simulink model "HopperRaibertSpeedGoat"  (R2025a)
settings: Solver=FixedStepAuto  StartTime=0.0  StopTime=inf  RelTol=1e-3
undefined symbols (not defined in the file): HS, IO291
libraries: aru_toolbox x3, speedgoatlib_IO291 x1, simulink x1
settings Model: Creator=Gavin  LastModifiedBy=user
settings SolverCC: ConcurrentTasks=on  PositivePriorityOrder=on  AutoInsertRateTranBlk=on
settings OptimizationCC: BlockReduction=off  OptimizeBlockIOStorage=off
settings DebuggingCC: TasksWithSamePriorityMsg=none
settings HardwareCC: ProdBitPerLong=64.0  ProdLongLongMode=on  ProdHWDeviceType=Intel->x86-64 (Linux 64)
settings RTWCC: SystemTargetFile=speedgoat.tlc  TemplateMakefile=slrealtime_default_tmf  Toolchain=Simulink Real-Time Toolchain  BuildConfiguration=Faster Runs  CodeExecutionProfiling=on  TargetLang=C++  Description=Speedgoat Real-Time Target Machine
settings SimulinkRealTimeTargetCC: SLRTFileLogMaxRuns=1.0  ExtModeMaxTrigDuration=10.0  ExtModeStaticAllocSize=1000000.0  ExtModeTransport=0.0  MultiwordLength=2048.0  DynamicStringBufferSize=256.0  PreserveMATLABNamespacesInGeneratedCode=on  SubcomponentCodeInterfacePackaging=Reusable function  MATLABClassNameForMDSCustomization=Simulink.SoftwareTarget.GRTCustomization  InstructionSetFMA=off  LogToMDFFile=off
settings ExplorerConfigSet: InternalSimMechanicsExplorerSettings="<ExplorerConfiguration><canonicalview>default</canonicalview><TilePanel><TileInfo><Tiles Columns=\"1\" Count=\"1\" Height=\"832\" Rows=\"1\" Width=\"1462\"><Row Weight=\"1\"/><Column Weight=\"1\"/><Tile Height=\"1\" Width=\"1\" X=\"0\" Y=\"0\"/></Tiles></TileInfo><SceneInfo><SceneViewer><IsThisViewStd><IsStandardView>off</IsStandardView><StandardViewName>Front</StandardViewName></IsThisViewStd><BGColor><R>1</R><G>1</G><B>1</B><A>1</A></BGColor><Camera><DoPerspective>on</DoPerspective><Position><X>-0.15165999999999999</X><Y>3.9971199999999998</Y><Z>0.85099999999999998</Z></Position><Center><X>0</X><Y>0</Y><Z>0.10100000000000001</Z></Center><Up><X>0.0069873130929931429</X><Y>-0.18415619748295364</Y><Z>0.98287215464899591</Z></Up><XLim>1.8977346774231529</XLim><YLim>1.8977346774231529</YLim><ViewLimDist>0.01</ViewLimDist></Camera></SceneViewer></SceneInfo></TilePanel><MechEditorPanel><GfxPanelCameraMap><MapElement CameraMLId=\"Camera1\" GfxPanelIndex=\"0\"/></GfxPanelCameraMap><Cameras><Camera><Id>Camera1</Id><Value><Name>FollowBot</Name><NativeCamera><PositionTrackingFeature>Subsystem.Half_Baleka_Simscape_WIP.Planarising_Boom.Center_to_CameraUp.F</PositionTrackingFeature><CenterTrackingFeature>Subsystem.Half_Baleka_Simscape_WIP.Planarising_Boom.Center_to_Camera.B</CenterTrackingFeature><UpVectorTrackingFeature>Subsystem.Half_Baleka_Simscape_WIP.Planarising_Boom.Center_to_Camera.B</UpVectorTrackingFeature><CenterTrackingOrigin>on</CenterTrackingOrigin><UpVectorTrackingDirection>+Y</UpVectorTrackingDirection></NativeCamera></Value></Camera></Cameras><VideoCreator><IncludeTiles>All</IncludeTiles><IncludeTime>on</IncludeTime><IncludeWorldFrame>off</IncludeWorldFrame><PlaybackSpeedRatio>1</PlaybackSpeedRatio><FrameRate>30</FrameRate><FrameSize>auto</FrameSize><VideoFormat>MotionJPEGAVI</VideoFormat></VideoCreator></MechEditorPanel><PlaybackSettings><PlaybackSpeedFactor>1</PlaybackSpeedFactor></PlaybackSettings></ExplorerConfiguration>"

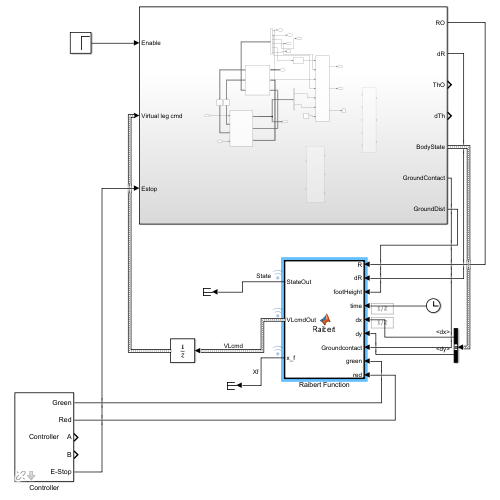
[thumbnail: Simulink's stored preview of the top-level diagram]
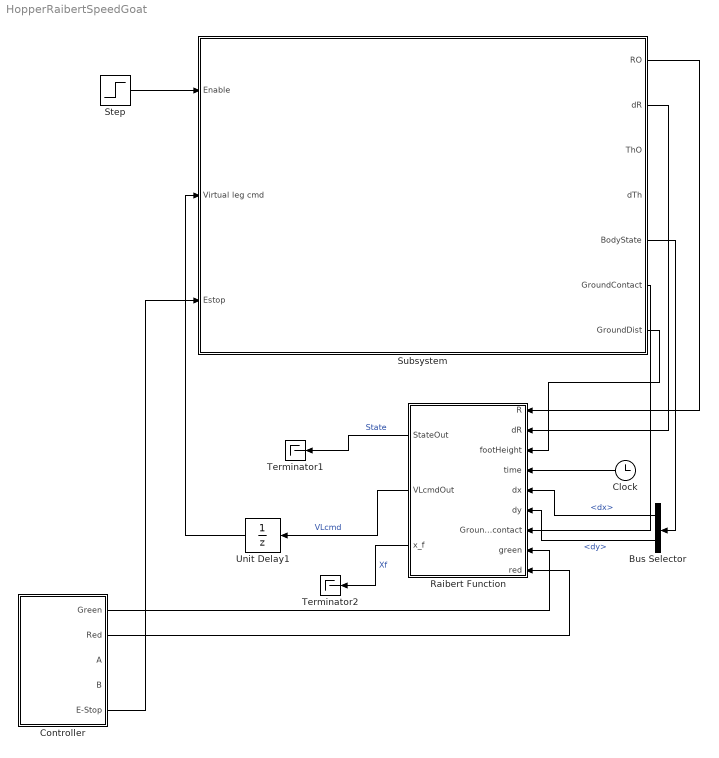
== system HopperRaibertSpeedGoat ==
  Bus Selector : BusSelector  OutputSignals=dx,dy
  Clock : Clock
  Controller : Subsystem  AncestorBlock=aru_toolbox/Controller
      mask Display:
      | disp('Controller');
      | port_label('output',1,'Green');
      | port_label('output',2,'Red');
      | port_label('output',3,'A');
      | port_label('output',4,'B');
      | port_label('output',5,'E-Stop');
  Raibert Function : MATLAB Function  TreatAsAtomicUnit=on
  Step : Step  Time=5  SampleTime=0
  Subsystem : Subsystem
  Terminator1 : Terminator
  Terminator2 : Terminator
  Unit Delay1 : UnitDelay  SampleTime=-1  HasFrameUpgradeWarning=on
  wires:
  Raibert Function/1(StateOut) -> Terminator1/1  "State"
  Subsystem/6(GroundContact) -> Raibert Function/7(Groundcontact)
  Subsystem/2(dR) -> Raibert Function/2(dR)
  Clock/1 -> Raibert Function/4(time)
  Subsystem/1(RO) -> Raibert Function/1(R)
  Subsystem/7(GroundDist) -> Raibert Function/3(footHeight)
  Subsystem/5(BodyState) -> Bus Selector/1
  Bus Selector/1 -> Raibert Function/5(dx)  "<dx>"
  Bus Selector/2 -> Raibert Function/6(dy)  "<dy>"
  Raibert Function/2(VLcmdOut) -> Unit Delay1/1  "VLcmd"
  Unit Delay1/1 -> Subsystem/2(Virtual leg cmd)
  Raibert Function/3(x_f) -> Terminator2/1  "Xf"
  Controller/5(E-Stop) -> Subsystem/3(Estop)
  Controller/1(Green) -> Raibert Function/8(green)
  Controller/2(Red) -> Raibert Function/9(red)
  Step/1 -> Subsystem/1(Enable)

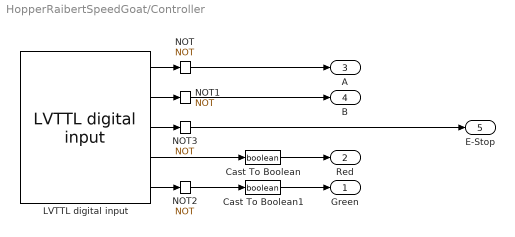
== system HopperRaibertSpeedGoat/Controller ==
  Cast To Boolean : DataTypeConversion  OutDataTypeStr=boolean  SaturateOnIntegerOverflow=off  RndMeth=Floor
  Cast To Boolean1 : DataTypeConversion  OutDataTypeStr=boolean  SaturateOnIntegerOverflow=off  RndMeth=Floor
  "LVTTL digital input " : speedgoatlib_IO291/LVTTL digital input   parModuleId=1  parSampleTime=-1  parPortConf=1 port for each active input channel  parDataType=Double  parPciSlot=-1  parTtlDiChannels=[1 2 3 4 5]  parModuleType=IO291-HS  parInternalModuleId=1
      settings: SourceProductName=IO291
  NOT{,1..3} (4 alike) : Logic  Operator=NOT  IconShape=distinctive  AllPortsSameDT=off  OutDataTypeStr=boolean
  Green : Outport
  Red : Outport  Port=2
  A : Outport  Port=3
  B : Outport  Port=4
  E-Stop : Outport  Port=5
  wires:
  Cast To Boolean1/1 -> Green/1
  Cast To Boolean/1 -> Red/1
  "LVTTL digital input "/4 -> Cast To Boolean/1
  "LVTTL digital input "/5 -> NOT2/1
  "LVTTL digital input "/1 -> NOT/1
  "LVTTL digital input "/2 -> NOT1/1
  NOT1/1 -> B/1
  "LVTTL digital input "/3 -> NOT3/1
  NOT/1 -> A/1
  NOT2/1 -> Cast To Boolean1/1
  NOT3/1 -> E-Stop/1

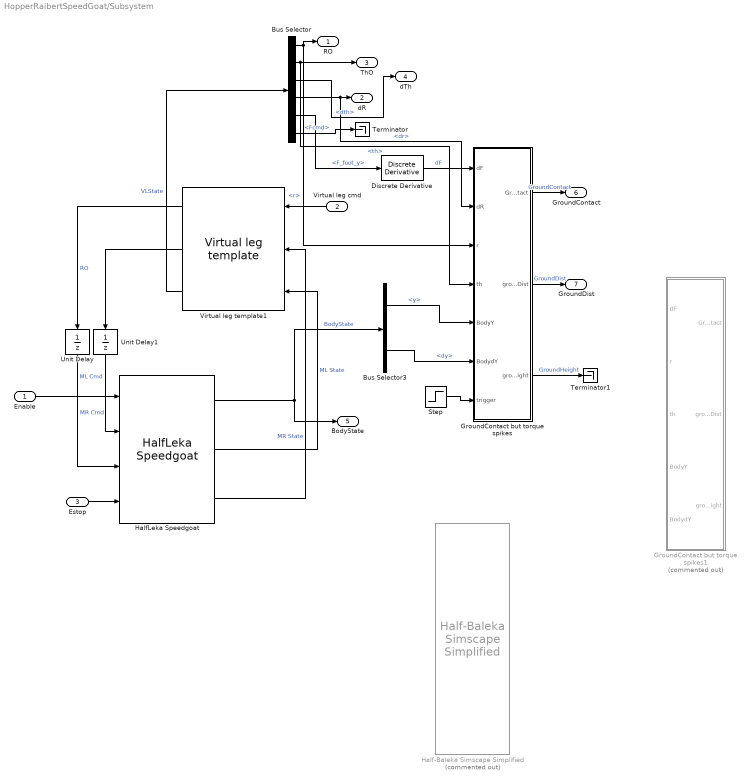
== system HopperRaibertSpeedGoat/Subsystem ==
  Enable : Inport
  Virtual leg cmd : Inport  Port=2  OutDataTypeStr=Bus: VLcmd
  Estop : Inport  Port=3
  Bus Selector : BusSelector  OutputSignals=r,th,dth,dr,F_foot_y,Fcmd
  Bus Selector3 : BusSelector  OutputSignals=y,dy
  Discrete Derivative : simulink/Discrete/Discrete Derivative  gainval=1.0  ICPrevScaledInput=0.0  OutMin=[]  OutMax=[]  OutDataType=fixdt(1, 16)  OutScaling=2^-10  DoSatur=off
  GroundContact but torque spikes : MATLAB Function  TreatAsAtomicUnit=on
  GroundContact but torque spikes1 : MATLAB Function  Commented=on  TreatAsAtomicUnit=on
  Half-Baleka Simscape Simplified : aru_toolbox/Baleka 2.5/Half-Baleka Simscape Simplified  Commented=on  communication_rate=1000  GravityBool=on  mu_s=1  mu_k=0.9  foot_k=1e5  foot_d=1e4  y_start=0.3  StartingMode=Zero (set Starting values manually)  LOffset=4.1  ROffset=-0.88
      settings: SourceProductName=ARU Toolbox
  HalfLeka Speedgoat : aru_toolbox/Baleka 2.5/HalfLeka Speedgoat  IDL=6  IDR=5  TscaleL=1.1986  TscaleR=1.2249
      link override Bus Creator2: Inputs=9
  Step : Step  Time=8  SampleTime=0
  Terminator : Terminator
  Terminator1 : Terminator
  Unit Delay : UnitDelay  SampleTime=-1  HasFrameUpgradeWarning=on
  Unit Delay1 : UnitDelay  SampleTime=-1  HasFrameUpgradeWarning=on
  Virtual leg template1 : aru_toolbox/Baleka 2.5/Virtual leg template  mx_tune=0.5543  cx_tune=-1.0796  my_tune=0.6663  cy_tune=-10.664
      settings: SourceProductName=ARU Toolbox
  RO : Outport
  dR : Outport  Port=2
  ThO : Outport  Port=3
  dTh : Outport  Port=4
  BodyState : Outport  Port=5
  GroundContact : Outport  Port=6
  GroundDist : Outport  Port=7
  wires:
  Bus Selector/6 -> Terminator/1  "<Fcmd>"
  Bus Selector/1 -> GroundContact but torque spikes/3(r), RO/1  "<r>"
  Unit Delay1/1 -> HalfLeka Speedgoat/2  "ML Cmd"
  Virtual leg cmd/1 -> Virtual leg template1/1
  Virtual leg template1/3 -> Bus Selector/1  "VLState"
  HalfLeka Speedgoat/3 -> Virtual leg template1/2  "MR State"
  HalfLeka Speedgoat/2 -> Virtual leg template1/3  "ML State"
  Virtual leg template1/1 -> Unit Delay/1  "RO"
  Bus Selector/2 -> ThO/1, GroundContact but torque spikes/4(th)  "<th>"
  Unit Delay/1 -> HalfLeka Speedgoat/3  "MR Cmd"
  HalfLeka Speedgoat/1 -> Bus Selector3/1, BodyState/1  "BodyState"
  Bus Selector/5 -> Discrete Derivative/1  "<F_foot_y>"
  GroundContact but torque spikes/1(GroundContact) -> GroundContact/1  "GroundContact"
  Virtual leg template1/2 -> Unit Delay1/1
  Bus Selector3/1 -> GroundContact but torque spikes/5(BodyY)  "<y>"
  Bus Selector3/2 -> GroundContact but torque spikes/6(BodydY)  "<dy>"
  GroundContact but torque spikes/3(groundHeight) -> Terminator1/1  "GroundHeight"
  Discrete Derivative/1 -> GroundContact but torque spikes/1(dF)  "dF"
  GroundContact but torque spikes/2(groundDist) -> GroundDist/1  "GroundDist"
  Step/1 -> GroundContact but torque spikes/7(trigger)
  Estop/1 -> HalfLeka Speedgoat/4
  Enable/1 -> HalfLeka Speedgoat/1
  Bus Selector/4 -> GroundContact but torque spikes/2(dR), dR/1  "<dr>"
  Bus Selector/3 -> dTh/1  "<dth>"

== matlab function HopperRaibertSpeedGoat/Raibert Function ==
  settings: sampleTime=0.001
  data: R input; StateOut output; dR input; footHeight input; time input; dx input; dy input; VLcmdOut output Bus: VLcmd; Groundcontact input; x_f output; green input; red input
function [StateOut, VLcmdOut, x_f]   = Raibert(R, dR,footHeight, time,dx, dy, Groundcontact, green, red)
    % Raibert hopping state machine
    persistent state landTime VLcmd x_f_des %dR
    % State variable
    % 0 = SETUP
    % 1 = FLIGHT
    % 2 = COMPRESSION
    % 3 = THRUST
    
    % Params:
    Ts = 0.25;
    Kdx = -0.01;
    dx_d = 2;


    x_f = dx*Ts/2 + Kdx*(dx - dx_d); % Foot placement
    % x_f = 0.1;
    
    if isempty(state)
        state = 0;
        x_f_des = 0;
        landTime = 99;
        % dR = 0;
        VLcmd.r_des = 0.45;
        VLcmd.dr_des =0;
        VLcmd.KPr = 1000;
        VLcmd.KDr =40;
        VLcmd.Fff =0;
        VLcmd.th_des = -pi/2;
        VLcmd.dth_des =0;
        VLcmd.KPth = 200;
        VLcmd.KDth = 5;
        VLcmd.Tff = 0;
        
    end

switch state
    case 0 % SETUP
        % Specific commands for first landing
        VLcmd.r_des = 0.25;
        VLcmd.dr_des =0;
        VLcmd.KPr = 1000;
        VLcmd.KDr =50;
        VLcmd.Fff =0;

        VLcmd.th_des = -pi/2 + asin(-0.07/0.25);
        VLcmd.KPth = 100;
        VLcmd.KDth = 20;
        % if Groundcontact % On foot touching ground go to COMPRESSION
        if green % wait for setup
            state = 4;
            landTime = time;
            x_f_des = 0.07;

        end
        if red
            state = 5;
        end
    case 1 % FLIGHT
        % Brace for impact with high-ish spring
        VLcmd.r_des = 0.45;
        VLcmd.dr_des =0;
        VLcmd.KPr = 600;
        VLcmd.KDr =20;
        VLcmd.Fff = 0;
        % Position leg for landing
        VLcmd.th_des = -pi/2 + asin(x_f/R);
        VLcmd.dth_des = 0;
        VLcmd.KPth = 100;
        VLcmd.KDth = 10;

        if Groundcontact % On foot touching ground go to COMPRESSION
            state = 2;
            landTime = time;
            x_f_des = x_f;
        end
        if red
            state = 5;
        end
    case 2 % COMPRESSION
        % Let spring compress
        VLcmd.r_des = 0.45;
        VLcmd.dr_des =0;
        VLcmd.KPr = 750;
        VLcmd.KDr =20;
        VLcmd.Fff = 0;
        % Servo hip
        VLcmd.th_des = -pi/2- asin(x_f_des/R); 
        VLcmd.dth_des = 0;%(dx*R - dR*R*sin(th))/(cos(th)*R^2);
        VLcmd.KPth = 250;
        VLcmd.KDth = 5;
        % When leg stops compressing (dR = 0) go to THRUST
        if (((time-landTime)>0.05)&&(dR>0)) 
            state = 3;
        end
        if red
            state = 5;
        end
    case 3 % THRUST
        % Apply upwards thrust force
        VLcmd.r_des = 0.6;
        VLcmd.dr_des =0;
        VLcmd.KPr = 1500;
        VLcmd.KDr =0;
        VLcmd.Fff = 0;% 2000;

        % Servo hip
        VLcmd.th_des = -pi/2 - asin(x_f_des/R); 
        VLcmd.dth_des = 0;%(dx*R - dR*R*sin(th))/(cos(th)*R^2);
        VLcmd.KPth = 400;
        VLcmd.KDth = 10;

        if ~Groundcontact%&&(dy>0))% ||((th1>3*pi/2)||(th2<-pi/2))
            state =1;
        end
        if red
            state = 5;
        end
    case 4 % StartingTHRUST
        % Apply upwards thrust force
        VLcmd.r_des = 0.6;
        VLcmd.dr_des =0;
        VLcmd.KPr = 1000;
        VLcmd.KDr =0;
        VLcmd.Fff = 0;% 2000;

        % Servo hip
        VLcmd.th_des = -pi/2 - asin(x_f_des/R); 
        VLcmd.dth_des = 0;%(dx*R - dR*R*sin(th))/(cos(th)*R^2);
        VLcmd.KPth = 600;
        VLcmd.KDth = 15;

        if ~Groundcontact%&&(dy>0))% ||((th1>3*pi/2)||(th2<-pi/2))
            state =1;
        end
        if red
            state = 5;
        end

    case 5 % HALT
        
        VLcmd.r_des = 0.45;
        VLcmd.dr_des =0;
        VLcmd.KPr = 900;
        VLcmd.KDr =10;
        VLcmd.Fff = 0;% 2000;

        % Servo hip
        VLcmd.th_des = -pi/2; 
        VLcmd.dth_des = 0;%(dx*R - dR*R*sin(th))/(cos(th)*R^2);
        VLcmd.KPth = 600;
        VLcmd.KDth = 10;

  

end
    VLcmdOut.r_des = VLcmd.r_des;
    VLcmdOut.dr_des = VLcmd.dr_des;
    VLcmdOut.KPr = VLcmd.KPr;
    VLcmdOut.KDr = VLcmd.KDr;
    VLcmdOut.Fff = VLcmd.Fff;

    VLcmdOut.th_des = VLcmd.th_des;
    VLcmdOut.dth_des = VLcmd.dth_des;
    VLcmdOut.KPth = VLcmd.KPth;
    VLcmdOut.KDth = VLcmd.KDth;
    VLcmdOut.Tff = VLcmd.Tff;

    StateOut = state;
end

== matlab function HopperRaibertSpeedGoat/Subsystem/GroundContact but torque spikes ==
  settings: sampleTime=0.001
  data: dF input; dR input; r input; th input; GroundContact output; BodyY input; groundDist output; groundHeight output; BodydY input; trigger input
function [GroundContact, groundDist, groundHeight]  = ImpactTorque(dF, dR, r, th, BodyY, BodydY, trigger)
        % need to see how IRL torque spikes work, but we can do a veeery
        % rough guestimate here:
        persistent GroundContactpers;
        persistent GroundHeight;
        if isempty(GroundContactpers)
            GroundContactpers = true;
            GroundHeight = 0;
        end
        if trigger >0
        %     GroundContactpers = true;
        %     GroundHeight = BodyY  +sin(th)*r;
        % end
        groundDist = BodyY + sin(th)*r;% - 0.004
            if ~GroundContactpers % Impact sensing for gnd
               if (dR<-1.2) && (BodydY <0) && (groundDist <0.07)
                GroundContactpers = true;
                GroundHeight = BodyY  +sin(th)*r; % - 0.004
               end
               groundDist=BodyY + sin(th)*r;
            else 
                % leg length calc for flight
                
                if BodydY >0
                    GroundContactpers = ~(groundDist>0.005+GroundHeight);
                end
            end

        else
            groundDist=BodyY + sin(th)*r;
            GroundHeight=BodyY + sin(th)*r;
        end
          
        GroundContact = GroundContactpers;
        groundHeight = GroundHeight;
end

== matlab function HopperRaibertSpeedGoat/Subsystem/GroundContact but torque spikes1 ==
  data: dF input; r input; th input; GroundContact output; BodyY input; groundDist output; groundHeight output; BodydY input
function [GroundContact, groundDist, groundHeight]  = ImpactTorque(dF,r, th, BodyY, BodydY)
        % need to see how IRL torque spikes work, but we can do a veeery
        % rough guestimate here:
        persistent GroundContactpers;
        persistent GroundHeight;
        if isempty(GroundContactpers)
            GroundContactpers = true;
            GroundHeight = 0;
        end

        if ~GroundContactpers % Impact sensing for gnd
           if (dF>3e4) && (BodydY <0)
            GroundContactpers = true;
            GroundHeight = BodyY  +sin(th)*r; % - 0.004
           end
           groundDist=BodyY + sin(th)*r;
        else 
            % leg length calc for flight
            groundDist = BodyY + sin(th)*r;% - 0.004
            if BodydY >0
                GroundContactpers = ~(groundDist>0.02+GroundHeight);
            end
        end
          
        GroundContact = GroundContactpers;
        groundHeight = GroundHeight;
end
